simulink library "PC_Simulator_Lib"  (Simulink 8.2)
settings: Solver=ode45  StartTime=0.0  StopTime=10.0  RelTol=1e-3
values from neighbouring files (symbols this model uses):
  data = [r1 r2 r3 r4 L1 L2 L3 L4]    [strasse_Bedatung_HNI_ITI.m]
  distSameLane = 60    [InitialisationsEnv.m]
  eng_speed = [0 60 120 180 240 300 360 420 480 540 600 660 ... (101 elements, 1x101)]    [engine_table.mat]    (also in motor_parameter_calc.m = omega)
  Heading_init = 0    [Start.m]
  inertiaLateral = 25*(radiusWheel)^2    (= 4.129024)    [Start.m]
  laneWidth = 3.6    [InitialisationsEnv.m]    (also in strasse_Bedatung_HNI_ITI.m)
  omega_engine = [0.000000 150.000000 500.000000 1000.000000 1500.000000 2000.000000 2500.000000 3000.000000 3500.000000 4000.000000 4500.000000 5000.000000 5500.000000 6000.000000]    [friction_tables.m]
  omega_max = 6000    [engine_table.mat]    (also in motor_parameter_calc.m)
  omega_wheel = [0 20 40 60 80 100 122 143.7 164]    [friction_tables.m]
  para_Fellow_8_Points = ADAS.Fellow_8_Points    [ADAS_parameters.m]
  position_start_x = [x1 x2 x3 x4 x5 x6 x7]    [strasse_Bedatung_HNI_ITI.m]
  position_start_y = [y1 y2 y3 y4 y5 y6 y7]    [strasse_Bedatung_HNI_ITI.m]
  rad3rdLine = 57.2    [InitialisationsEnv.m]    (also in strasse_Bedatung_HNI_ITI.m)
  radiusWheel = 16*2.54/100    (= 0.4064)    [Start.m]
  s_values = [S1 S2 S3 S4 S5 S6 S7]    [strasse_Bedatung_HNI_ITI.m]
  segmentLimits = [segment1EndThirdLine                   segment2EndThirdLine                   segment3EndThirdLine                   segment4EndThirdLine                   segment5EndThirdLine                   segment6EndThirdLine                   segment7EndThirdLine                   segment8EndThirdLine                   ]    [InitialisationsEnv.m]    (also in strasse_Bedatung_HNI_ITI.m)
  setPosT = [-1.8 -5.4 -1.8 -5.4 -1.8 -5.4 -1.8 -5.4 -1.8 -5.4]    [InitialisationsEnv.m]
  torque = [297.089227105 300.997600937 304.800343044 308.497453426 312.088932082 315.574779014 318.95499422 322.229577701 325.398529457 328.461849487 331.419537793 334.271594373 ... (101 elements, 1x101)]    [engine_table.mat]    (also in motor_parameter_calc.m = g)
  Torque_lost = [0.000000 -8.777780 -15.000000 -26.800000 -29.600000 -32.700000 -35.900000 -39.300000 -42.800000 -46.500000 -50.300000 -54.300000 -58.500000 -62.800000 ]*0.6    [friction_tables.m]
  Torque_lost_wheel = [0.8 0.8 0.75 0.7 0.4 0.3 0.2 0.07 0.07]*0.2    [friction_tables.m]
  X_init = 0    [Start.m]
  Y_init = 1.8    [Start.m]
  Z_init = 0    [Start.m]
undefined symbols (not defined in the file or in its folder): Acc_Pedal, ADAS, Brake_Pedal, Joystick, Newton, Para, Raphson, Standard_Devices, Steering_Wheel_Angle, UDP_Protocol
libraries: simulink x43, rtwinlib x7, dspnetwork x2, simulink_extras x1, vrlib x1
(part 4 of 13)

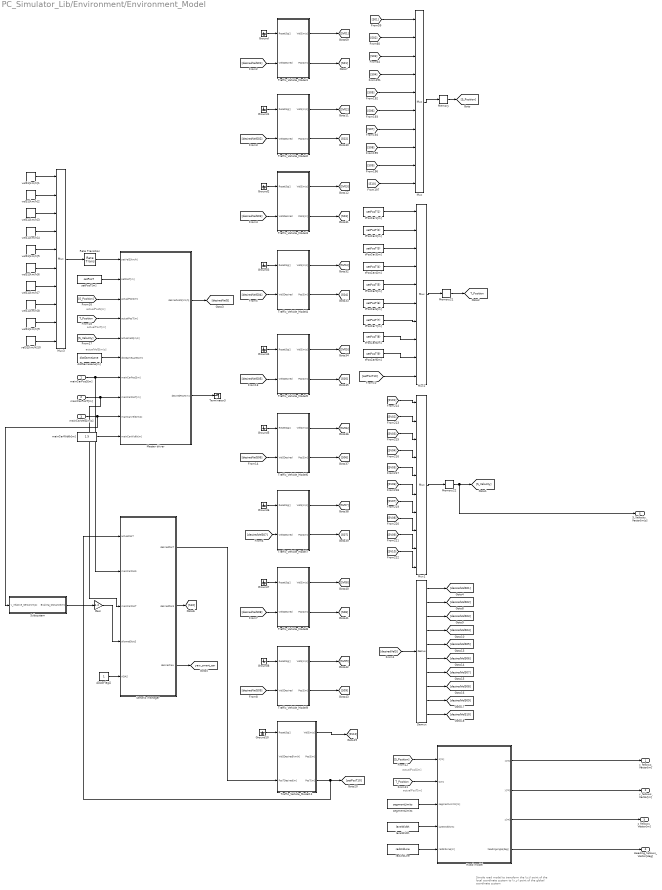
== system PC_Simulator_Lib/Environment/Environment_Model ==
  note: actualPosS[m]
  note: actualPosT[m]
  note: actualVelS[m/s]
  note: Simple road model to transform the (s,t) point of the
      | local coordinate system to (x,y) point of the global
      | coordinate system
  note: actualPosT[m]
  note: actualPosS[m]
  mainCarPosS[m] : Inport
  mainCarPosT[m] : Inport  Port=2
  mainCarVelS[m/s] : Inport  Port=3
  ADASFlag[] : Constant
  Demux : Demux  Outputs=10
  Gain : Gain  Gain=1.2
  Ground{,1..8,10} (10 alike) : Ground
  Master driver : Subsystem
  Memory : Memory
  Memory21 : Memory
  Memory22 : Memory
  Mux{,1..3} (4 alike) : Mux  Inputs=10
  Rate Transition : RateTransition
  Road model : Subsystem  Description=Simple road model to transform the (s,t) point of the local coordinate system to (x,y) point of the global coordinate system
  Senario manager : MATLAB Function  TreatAsAtomicUnit=on
  Subsystem : Subsystem
  Terminator3 : Terminator
  Traffic_Vehicle_Model1 : Subsystem
  Traffic_Vehicle_Model11 : Subsystem
  Traffic_Vehicle_Model2 : Subsystem
  Traffic_Vehicle_Model3 : Subsystem
  Traffic_Vehicle_Model4 : Subsystem
  Traffic_Vehicle_Model5 : Subsystem
  Traffic_Vehicle_Model6 : Subsystem
  Traffic_Vehicle_Model7 : Subsystem
  Traffic_Vehicle_Model8 : Subsystem
  Traffic_Vehicle_Model9 : Subsystem
  distSameLane[m] : Constant  Value=distSameLane
  laneWidth : Constant  Value=laneWidth
  mainCarWidth[m] : Constant  Value=1.5
  rad3rdLine : Constant  Value=rad3rdLine
  segmentLimits : Constant  Value=segmentLimits
  setPosT[m] : Constant  Value=setPosT
  tPosCar1[m] : Constant  Value=setPosT(1)
  tPosCar2[m] : Constant  Value=setPosT(2)
  tPosCar3[m] : Constant  Value=setPosT(3)
  tPosCar4[m] : Constant  Value=setPosT(4)
  tPosCar5[m] : Constant  Value=setPosT(5)
  tPosCar6[m] : Constant  Value=setPosT(6)
  tPosCar7[m] : Constant  Value=setPosT(7)
  tPosCar8[m] : Constant  Value=setPosT(8)
  tPosCar9[m] : Constant  Value=setPosT(9)
  velS1[km/h]1 : UniformRandomNumber  Minimum=0  Maximum=100  Seed=40  SampleTime=30
  velS1[km/h]{2..10} (9 alike) : UniformRandomNumber  Minimum=0  Maximum=100  SampleTime=30
  x_fellows_Vector[m] : Outport
  y_fellows_Vector[m] : Outport  Port=2
  z_fellows_Vector[m] : Outport  Port=3
  Heading_fellows_Vector[deg] : Outport  Port=4
  S_Velocity_Vector[m|s] : Outport  Port=5
  tag scope: T_Position=global, yaw_smart_car=global
  wires:
  [setPosT10] -> Mux2/10
  tPosCar9[m]/1 -> Mux2/9
  tPosCar8[m]/1 -> Mux2/8
  tPosCar7[m]/1 -> Mux2/7
  tPosCar3[m]/1 -> Mux2/3
  tPosCar4[m]/1 -> Mux2/4
  tPosCar1[m]/1 -> Mux2/1
  tPosCar2[m]/1 -> Mux2/2
  tPosCar6[m]/1 -> Mux2/6
  tPosCar5[m]/1 -> Mux2/5
  [S05] -> Mux/5
  [S08] -> Mux/8
  [S06] -> Mux/6
  [S07] -> Mux/7
  [S09] -> Mux/9
  [S10] -> Mux/10
  [S03] -> Mux/3
  [S04] -> Mux/4
  [S02] -> Mux/2
  [S01] -> Mux/1
  Gain/1 -> Senario manager/4(allowedDistS)
  Senario manager/1(desiredPosT) -> Traffic_Vehicle_Model11/3(PosTDesired[m])
  mainCarPosS[m]/1 -> Senario manager/2(mainCarPosS), Master driver/7(mainCarPosS[m])
  Subsystem/1(Braking_Distance[m]) -> Gain/1
  Senario manager/3(desiredYaw) -> [yaw_smart_car]
  Senario manager/2(desiredPosS) -> [S10]
  ADASFlag[]/1 -> Senario manager/5(ADAS)
  Traffic_Vehicle_Model11/3(PosT[m]) -> [setPosT10], Senario manager/1(actualPosT)
  mainCarPosT[m]/1 -> Master driver/8(mainCarPosT[m]), Senario manager/3(mainCarPosT)
  Traffic_Vehicle_Model11/1(VelS[m/s]) -> [SV10]
  Ground10/1 -> Traffic_Vehicle_Model11/1(ResetSig[])
  setPosT[m]/1 -> Master driver/2(setPosT[m])
  Master driver/2(desiredPosT[m]) -> Terminator3/1
  Mux/1 -> Memory/1
  Memory/1 -> [S_Position]
  Mux2/1 -> Memory21/1
  Memory21/1 -> [T_Position]
  Mux1/1 -> Memory22/1
  Memory22/1 -> S_Velocity_Vector[m|s]/1, [S_Velocity]
  [SV01] -> Mux1/1
  [SV02] -> Mux1/2
  [SV03] -> Mux1/3
  [SV04] -> Mux1/4
  [SV05] -> Mux1/5
  [SV06] -> Mux1/6
  [SV07] -> Mux1/7
  [SV08] -> Mux1/8
  [SV09] -> Mux1/9
  [SV10] -> Mux1/10
  [S_Position] -> Master driver/3(actualPosS[m])
  [T_Position] -> Master driver/4(actualPosT[m])
  [S_Velocity] -> Master driver/5(actualVelS[m/s])
  distSameLane[m]/1 -> Master driver/6(distSameLanes[m])
  Mux3/1 -> Rate Transition/1
  Master driver/1(desiredVelS[km/h]) -> [desiredVelS]
  [desiredVelS] -> Demux/1
  Demux/1 -> [desiredVelS01]
  Demux/2 -> [desiredVelS02]
  Demux/3 -> [desiredVelS03]
  Demux/4 -> [desiredVelS04]
  Demux/5 -> [desiredVelS05]
  Demux/6 -> [desiredVelS06]
  Demux/7 -> [desiredVelS07]
  Demux/8 -> [desiredVelS08]
  Demux/9 -> [desiredVelS09]
  Demux/10 -> [desiredVelS10]
  Ground/1 -> Traffic_Vehicle_Model1/1(ResetSig[])
  Traffic_Vehicle_Model1/2(PosS[m]) -> [S01]
  Traffic_Vehicle_Model1/1(VelS[m/s]) -> [SV01]
  [desiredVelS01] -> Traffic_Vehicle_Model1/2(VelSDesired)
  Ground1/1 -> Traffic_Vehicle_Model2/1(ResetSig[])
  Traffic_Vehicle_Model2/2(PosS[m]) -> [S02]
  Traffic_Vehicle_Model2/1(VelS[m/s]) -> [SV02]
  [desiredVelS02] -> Traffic_Vehicle_Model2/2(VelSDesired)
  Ground2/1 -> Traffic_Vehicle_Model3/1(ResetSig[])
  Traffic_Vehicle_Model3/2(PosS[m]) -> [S03]
  Traffic_Vehicle_Model3/1(VelS[m/s]) -> [SV03]
  [desiredVelS03] -> Traffic_Vehicle_Model3/2(VelSDesired)
  Ground3/1 -> Traffic_Vehicle_Model4/1(ResetSig[])
  Traffic_Vehicle_Model4/2(PosS[m]) -> [S04]
  Traffic_Vehicle_Model4/1(VelS[m/s]) -> [SV04]
  [desiredVelS04] -> Traffic_Vehicle_Model4/2(VelSDesired)
  Ground4/1 -> Traffic_Vehicle_Model5/1(ResetSig[])
  Traffic_Vehicle_Model5/2(PosS[m]) -> [S05]
  Traffic_Vehicle_Model5/1(VelS[m/s]) -> [SV05]
  [desiredVelS05] -> Traffic_Vehicle_Model5/2(VelSDesired)
  Ground5/1 -> Traffic_Vehicle_Model6/1(ResetSig[])
  Traffic_Vehicle_Model6/2(PosS[m]) -> [S06]
  Traffic_Vehicle_Model6/1(VelS[m/s]) -> [SV06]
  [desiredVelS06] -> Traffic_Vehicle_Model6/2(VelSDesired)
  Ground6/1 -> Traffic_Vehicle_Model7/1(ResetSig[])
  Traffic_Vehicle_Model7/2(PosS[m]) -> [S07]
  Traffic_Vehicle_Model7/1(VelS[m/s]) -> [SV07]
  [desiredVelS07] -> Traffic_Vehicle_Model7/2(VelSDesired)
  Ground7/1 -> Traffic_Vehicle_Model8/1(ResetSig[])
  Traffic_Vehicle_Model8/2(PosS[m]) -> [S08]
  Traffic_Vehicle_Model8/1(VelS[m/s]) -> [SV08]
  [desiredVelS08] -> Traffic_Vehicle_Model8/2(VelSDesired)
  Ground8/1 -> Traffic_Vehicle_Model9/1(ResetSig[])
  Traffic_Vehicle_Model9/2(PosS[m]) -> [S09]
  Traffic_Vehicle_Model9/1(VelS[m/s]) -> [SV09]
  [desiredVelS09] -> Traffic_Vehicle_Model9/2(VelSDesired)
  Road model/4(headingAngle[deg]) -> Heading_fellows_Vector[deg]/1
  Road model/2(y[m]) -> y_fellows_Vector[m]/1
  Road model/1(x[m]) -> x_fellows_Vector[m]/1
  Road model/3(z[m]) -> z_fellows_Vector[m]/1
  velS1[km/h]2/1 -> Mux3/2
  velS1[km/h]4/1 -> Mux3/4
  [S_Position] -> Road model/1(s[m])
  [T_Position] -> Road model/2(t[m])
  velS1[km/h]1/1 -> Mux3/1
  rad3rdLine/1 -> Road model/5(rad3rdLine[m])
  laneWidth/1 -> Road model/4(laneWidth[m])
  mainCarWidth[m]/1 -> Master driver/10(mainCarWidth[m])
  segmentLimits/1 -> Road model/3(segmentLimits[m])
  velS1[km/h]9/1 -> Mux3/9
  velS1[km/h]8/1 -> Mux3/8
  velS1[km/h]3/1 -> Mux3/3
  velS1[km/h]7/1 -> Mux3/7
  velS1[km/h]6/1 -> Mux3/6
  Rate Transition/1 -> Master driver/1(setVelS[km/h])
  velS1[km/h]5/1 -> Mux3/5
  velS1[km/h]10/1 -> Mux3/10
  mainCarVelS[m/s]/1 -> Master driver/9(mainCarVelS[m/s]), Subsystem/1(v_relative_Sensor[m|s])

== system PC_Simulator_Lib/Environment/Maping_Input  ==
  Feedback : Inport
  Bus Selector10 : BusSelector  OutputSignals=Vehicle_Dynamics.position_CoG.x_CoG[m],Vehicle_Dynamics.position_CoG.y_CoG[m],Vehicle_Dynamics.Vx_COG[m|s]
  Gain : Gain  Gain=180/pi
  Strasse_xy : Subsystem
  mainCarPosS[m] : Outport
  mainCarPosT[m] : Outport  Port=2
  mainCarVelS[m/s] : Outport  Port=3
  Heating_Angle_Road_under_VUT[deg] : Outport  Port=4
  wires:
  Bus Selector10/1 -> Strasse_xy/1(x[m])  "<x_CoG[m]>"
  Bus Selector10/2 -> Strasse_xy/2(y[m])  "<y_CoG[m]>"
  Strasse_xy/2(t[m]) -> mainCarPosT[m]/1  "t_VUT[m]"
  Strasse_xy/1(s[m]) -> mainCarPosS[m]/1  "s_VUT[m]"
  Feedback/1 -> Bus Selector10/1
  Bus Selector10/3 -> mainCarVelS[m/s]/1  "<Vx_COG[m|s]>"
  Strasse_xy/3(Heading_angle[rad]) -> Gain/1
  Gain/1 -> Heating_Angle_Road_under_VUT[deg]/1

== system PC_Simulator_Lib/Environment/Maping_Output  ==
  x_fellows_Vector[m] : Inport
  y_fellows_Vector[m] : Inport  Port=2
  z_fellows_Vector[m] : Inport  Port=3
  Heading_fellows_Vector[deg] : Inport  Port=4
  S_Velocity_Vector[m|s] : Inport  Port=5
  T_VUT[m] : Inport  Port=6
  Heating_Angle_Road_under_VUT[deg] : Inport  Port=7
  Bus Creator : BusCreator  Inputs=11
  Bus Creator{1,3..11} (10 alike) : BusCreator  Inputs=5
  Bus Creator2 : BusCreator  Inputs=2
  Bus Selector : BusSelector  OutputSignals=x_fellows_vector.x_fellow1[m],y_fellows_vector.y_fellow1[m],z_fellows_vector.z_fellow1[m],Heading_fellows_vector.Heading_fellow1[deg],velocity_fellows_vector[m|s].velocity_fellow1[m|s]
  Bus Selector1 : BusSelector  OutputSignals=x_fellows_vector.x_fellow2[m],y_fellows_vector.y_fellow2[m],z_fellows_vector.z_fellow2[m],Heading_fellows_vector.Heading_fellow2[deg],velocity_fellows_vector[m|s].velocity_fellow2[m|s]
  Bus Selector2 : BusSelector  OutputSignals=x_fellows_vector.x_fellow3[m],y_fellows_vector.y_fellow3[m],z_fellows_vector.z_fellow3[m],Heading_fellows_vector.Heading_fellow3[deg],velocity_fellows_vector[m|s].velocity_fellow3[m|s]
  Bus Selector3 : BusSelector  OutputSignals=x_fellows_vector.x_fellow4[m],y_fellows_vector.y_fellow4[m],z_fellows_vector.z_fellow4[m],Heading_fellows_vector.Heading_fellow4[deg],velocity_fellows_vector[m|s].velocity_fellow4[m|s]
  Bus Selector4 : BusSelector  OutputSignals=x_fellows_vector.x_fellow5[m],y_fellows_vector.y_fellow5[m],z_fellows_vector.z_fellow5[m],Heading_fellows_vector.Heading_fellow5[deg],velocity_fellows_vector[m|s].velocity_fellow5[m|s]
  Bus Selector5 : BusSelector  OutputSignals=x_fellows_vector.x_fellow6[m],y_fellows_vector.y_fellow6[m],z_fellows_vector.z_fellow6[m],Heading_fellows_vector.Heading_fellow6[deg],velocity_fellows_vector[m|s].velocity_fellow6[m|s]
  Bus Selector6 : BusSelector  OutputSignals=x_fellows_vector.x_fellow7[m],y_fellows_vector.y_fellow7[m],z_fellows_vector.z_fellow7[m],Heading_fellows_vector.Heading_fellow7[deg],velocity_fellows_vector[m|s].velocity_fellow7[m|s]
  Bus Selector7 : BusSelector  OutputSignals=x_fellows_vector.x_fellow8[m],y_fellows_vector.y_fellow8[m],z_fellows_vector.z_fellow8[m],Heading_fellows_vector.Heading_fellow8[deg],velocity_fellows_vector[m|s].velocity_fellow8[m|s]
  Bus Selector8 : BusSelector  OutputSignals=x_fellows_vector.x_fellow9[m],y_fellows_vector.y_fellow9[m],z_fellows_vector.z_fellow9[m],Heading_fellows_vector.Heading_fellow9[deg],velocity_fellows_vector[m|s].velocity_fellow9[m|s]
  Bus Selector9 : BusSelector  OutputSignals=x_fellows_vector.x_fellow10[m],y_fellows_vector.y_fellow10[m],z_fellows_vector.z_fellow10[m],Heading_fellows_vector.Heading_fellow10[deg],velocity_fellows_vector[m|s].velocity_fellow10[m|s]
  Subsystem : Subsystem
  Out1 : Outport
  wires:
  Bus Creator/1 -> Out1/1  "Environment"
  Bus Selector/2 -> Bus Creator1/2  "<y_fellow1[m]>"
  Bus Selector/1 -> Bus Creator1/1  "<x_fellow1[m]>"
  Bus Selector/4 -> Bus Creator1/4  "<Heading_fellow1[deg]>"
  Bus Creator1/1 -> Bus Creator/2  "fellow_car_1"
  Bus Creator2/1 -> Bus Creator/1  "Main_Vehicle"
  Bus Selector/3 -> Bus Creator1/3  "<z_fellow1[m]>"
  x_fellows_Vector[m]/1 -> Subsystem/1(x_fellows_Vector[m])
  y_fellows_Vector[m]/1 -> Subsystem/2(y_fellows_Vector[m])
  z_fellows_Vector[m]/1 -> Subsystem/3(z_fellows_Vector[m])
  Heading_fellows_Vector[deg]/1 -> Subsystem/4(Heading_fellows_Vector[deg])
  Subsystem/1(Fellows_Pos_Oriantation_Bus) -> Bus Selector9/1, Bus Selector8/1, Bus Selector7/1, Bus Selector6/1, Bus Selector5/1, Bus Selector4/1, Bus Selector3/1, Bus Selector2/1, Bus Selector1/1, Bus Selector/1
  Bus Selector1/2 -> Bus Creator3/2  "<y_fellow2[m]>"
  Bus Selector1/1 -> Bus Creator3/1  "<x_fellow2[m]>"
  Bus Selector1/4 -> Bus Creator3/4  "<Heading_fellow2[deg]>"
  Bus Creator3/1 -> Bus Creator/3  "fellow_car_2"
  Bus Selector1/3 -> Bus Creator3/3  "<z_fellow2[m]>"
  Bus Selector2/2 -> Bus Creator4/2  "<y_fellow3[m]>"
  Bus Selector2/1 -> Bus Creator4/1  "<x_fellow3[m]>"
  Bus Selector2/4 -> Bus Creator4/4  "<Heading_fellow3[deg]>"
  Bus Creator4/1 -> Bus Creator/4  "fellow_car_3"
  Bus Selector2/3 -> Bus Creator4/3  "<z_fellow3[m]>"
  Bus Selector3/2 -> Bus Creator5/2  "<y_fellow4[m]>"
  Bus Selector3/1 -> Bus Creator5/1  "<x_fellow4[m]>"
  Bus Selector3/4 -> Bus Creator5/4  "<Heading_fellow4[deg]>"
  Bus Creator5/1 -> Bus Creator/5  "fellow_car_4"
  Bus Selector3/3 -> Bus Creator5/3  "<z_fellow4[m]>"
  Bus Selector4/2 -> Bus Creator6/2  "<y_fellow5[m]>"
  Bus Selector4/1 -> Bus Creator6/1  "<x_fellow5[m]>"
  Bus Selector4/4 -> Bus Creator6/4  "<Heading_fellow5[deg]>"
  Bus Creator6/1 -> Bus Creator/6  "fellow_car_5"
  Bus Selector4/3 -> Bus Creator6/3  "<z_fellow5[m]>"
  Bus Creator7/1 -> Bus Creator/7  "fellow_car_6"
  Bus Creator8/1 -> Bus Creator/8  "fellow_car_7"
  Bus Creator9/1 -> Bus Creator/9  "fellow_car_8"
  Bus Creator10/1 -> Bus Creator/10  "fellow_car_9"
  Bus Creator11/1 -> Bus Creator/11  "fellow_car_10"
  Bus Selector5/3 -> Bus Creator7/3  "<z_fellow6[m]>"
  Bus Selector5/4 -> Bus Creator7/4  "<Heading_fellow6[deg]>"
  Bus Selector5/2 -> Bus Creator7/2  "<y_fellow6[m]>"
  Bus Selector5/1 -> Bus Creator7/1  "<x_fellow6[m]>"
  Bus Selector6/2 -> Bus Creator8/2  "<y_fellow7[m]>"
  Bus Selector6/4 -> Bus Creator8/4  "<Heading_fellow7[deg]>"
  Bus Selector6/1 -> Bus Creator8/1  "<x_fellow7[m]>"
  Bus Selector6/3 -> Bus Creator8/3  "<z_fellow7[m]>"
  Bus Selector7/2 -> Bus Creator9/2  "<y_fellow8[m]>"
  Bus Selector7/1 -> Bus Creator9/1  "<x_fellow8[m]>"
  Bus Selector7/3 -> Bus Creator9/3  "<z_fellow8[m]>"
  Bus Selector7/4 -> Bus Creator9/4  "<Heading_fellow8[deg]>"
  Bus Selector8/2 -> Bus Creator10/2  "<y_fellow9[m]>"
  Bus Selector8/1 -> Bus Creator10/1  "<x_fellow9[m]>"
  Bus Selector8/4 -> Bus Creator10/4  "<Heading_fellow9[deg]>"
  Bus Selector8/3 -> Bus Creator10/3  "<z_fellow9[m]>"
  Bus Selector9/4 -> Bus Creator11/4  "<Heading_fellow10[deg]>"
  Bus Selector9/3 -> Bus Creator11/3  "<z_fellow10[m]>"
  Bus Selector9/1 -> Bus Creator11/1  "<x_fellow10[m]>"
  Bus Selector9/2 -> Bus Creator11/2  "<y_fellow10[m]>"
  T_VUT[m]/1 -> Bus Creator2/1
  S_Velocity_Vector[m|s]/1 -> Subsystem/5(S_Velocity_Vector[m|s])
  Bus Selector/5 -> Bus Creator1/5  "<velocity_fellow1[m|s]>"
  Bus Selector1/5 -> Bus Creator3/5  "<velocity_fellow2[m|s]>"
  Bus Selector2/5 -> Bus Creator4/5  "<velocity_fellow3[m|s]>"
  Bus Selector3/5 -> Bus Creator5/5  "<velocity_fellow4[m|s]>"
  Bus Selector4/5 -> Bus Creator6/5  "<velocity_fellow5[m|s]>"
  Bus Selector5/5 -> Bus Creator7/5  "<velocity_fellow6[m|s]>"
  Bus Selector6/5 -> Bus Creator8/5  "<velocity_fellow7[m|s]>"
  Bus Selector7/5 -> Bus Creator9/5  "<velocity_fellow8[m|s]>"
  Bus Selector8/5 -> Bus Creator10/5  "<velocity_fellow9[m|s]>"
  Bus Selector9/5 -> Bus Creator11/5  "<velocity_fellow10[m|s]>"
  Heating_Angle_Road_under_VUT[deg]/1 -> Bus Creator2/2  "Heating_Angle_Road_under_VUT[deg]"

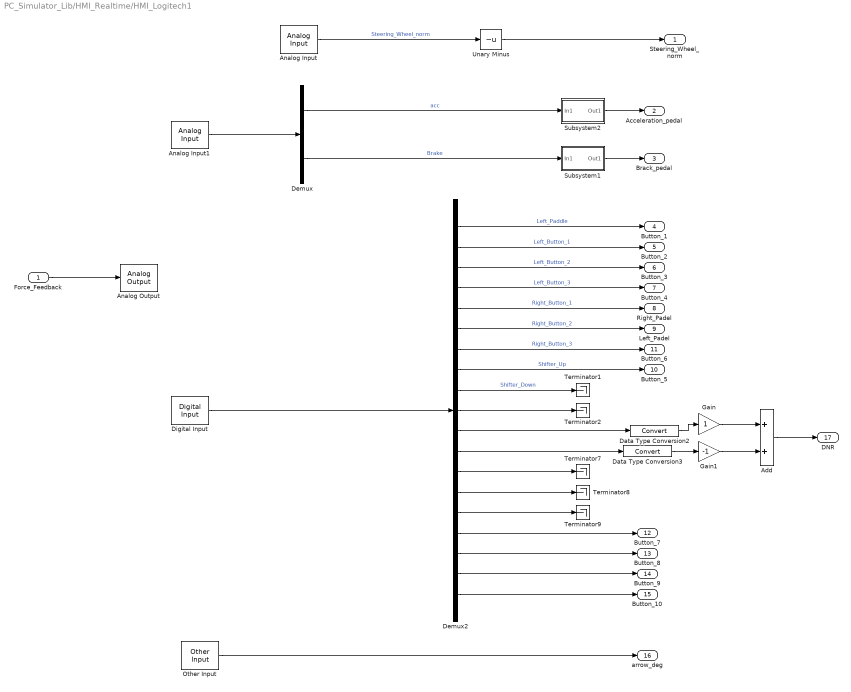
== system PC_Simulator_Lib/HMI_Realtime/HMI_Logitech1 ==
  Force_Feedback : Inport
  Add : Sum
  Analog Input : rtwinlib/Analog Input  SampleTime=-1  MaxMissedTicks=[]  ShowMissedTicks=off  YieldWhenWaiting=off  DrvName=Standard_Devices/Joystick  DrvAddress=1  DrvOptions=zeros(1,0)  Channels=1  RangeMode=2  VoltRange=1  DataType=1
      settings: AttributesFormatString=Standard Devices\nJoystick [1h]
  Analog Input1 : rtwinlib/Analog Input  SampleTime=-1  MaxMissedTicks=[]  ShowMissedTicks=off  YieldWhenWaiting=off  DrvName=Standard_Devices/Joystick  DrvAddress=1  DrvOptions=zeros(1,0)  Channels=2:3  RangeMode=3  VoltRange=1  DataType=1
      settings: AttributesFormatString=Standard Devices\nJoystick [1h]
  Analog Output : rtwinlib/Analog Output  SampleTime=0.001  MaxMissedTicks=[]  ShowMissedTicks=off  YieldWhenWaiting=off  DrvName=Standard_Devices/Joystick  DrvAddress=1  DrvOptions=zeros(1,0)  Channels=1  RangeMode=1  VoltRange=1  InitialValue=[]  FinalValue=[]
      settings: AttributesFormatString=Standard Devices\nJoystick [1h]
  Data Type Conversion2 : DataTypeConversion
  Data Type Conversion3 : DataTypeConversion
  Demux : Demux  Outputs=2
  Demux2 : Demux  Outputs=19
  Digital Input : rtwinlib/Digital Input  SampleTime=-1  MaxMissedTicks=[]  ShowMissedTicks=off  YieldWhenWaiting=off  DrvName=Standard_Devices/Joystick  DrvAddress=1  DrvOptions=zeros(1,0)  Channels=1:19  BitMode=1  DataType=1
      settings: AttributesFormatString=Standard Devices\nJoystick [1h]
  Gain : Gain
  Gain1 : Gain  Gain=-1
  Other Input : rtwinlib/Other Input  SampleTime=-1  MaxMissedTicks=[]  ShowMissedTicks=off  YieldWhenWaiting=off  DrvName=Standard_Devices/Joystick  DrvAddress=1  DrvOptions=zeros(1,0)  Channels=1  OptParam=0  DataType=1
      settings: AttributesFormatString=Standard Devices\nJoystick [1h]
  Subsystem1 : Subsystem
  Subsystem2 : Subsystem
  Terminator{1..2,7..9} (5 alike) : Terminator
  Unary Minus : UnaryMinus
  Steering_Wheel_norm : Outport
  Acceleration_pedal : Outport  Port=2
  Brack_pedal : Outport  Port=3
  Button_1 : Outport  Port=4
  Button_2 : Outport  Port=5
  Button_3 : Outport  Port=6
  Button_4 : Outport  Port=7
  Right_Padel : Outport  Port=8
  Left_Padel : Outport  Port=9
  Button_5 : Outport  Port=10
  Button_6 : Outport  Port=11
  Button_7 : Outport  Port=12
  Button_8 : Outport  Port=13
  Button_9 : Outport  Port=14
  Button_10 : Outport  Port=15
  arrow_deg : Outport  Port=16
  DNR : Outport  Port=17
  wires:
  Demux2/12 -> Data Type Conversion3/1
  Demux2/11 -> Data Type Conversion2/1
  Demux2/10 -> Terminator2/1
  Demux2/9 -> Terminator1/1  "Shifter_Down"
  Digital Input/1 -> Demux2/1
  Demux/1 -> Subsystem2/1(In1)  "acc"
  Demux/2 -> Subsystem1/1(In1)  "Brake"
  Analog Input/1 -> Unary Minus/1  "Steering_Wheel_norm"
  Subsystem2/1(Out1) -> Acceleration_pedal/1
  Subsystem1/1(Out1) -> Brack_pedal/1
  Demux2/1 -> Button_1/1  "Left_Paddle"
  Demux2/2 -> Button_2/1  "Left_Button_1"
  Demux2/3 -> Button_3/1  "Left_Button_2"
  Demux2/4 -> Button_4/1  "Left_Button_3"
  Demux2/5 -> Right_Padel/1  "Right_Button_1"
  Demux2/6 -> Left_Padel/1  "Right_Button_2"
  Demux2/7 -> Button_6/1  "Right_Button_3"
  Demux2/8 -> Button_5/1  "Shifter_Up"
  Demux2/16 -> Button_7/1
  Demux2/17 -> Button_8/1
  Demux2/18 -> Button_9/1
  Demux2/19 -> Button_10/1
  Other Input/1 -> arrow_deg/1
  Unary Minus/1 -> Steering_Wheel_norm/1
  Gain/1 -> Add/1
  Gain1/1 -> Add/2
  Add/1 -> DNR/1
  Data Type Conversion2/1 -> Gain/1
  Data Type Conversion3/1 -> Gain1/1
  Demux2/13 -> Terminator7/1
  Demux2/14 -> Terminator8/1
  Demux2/15 -> Terminator9/1
  Analog Input1/1 -> Demux/1
  Force_Feedback/1 -> Analog Output/1

== system PC_Simulator_Lib/HMI_Realtime/Maping_Output ==
  Steering_wheel_norm : Inport
  Acc_Pedal_norm : Inport  Port=2
  Brake_Pedal_norm : Inport  Port=3
  ACC_Plus : Inport  Port=4
  ACC_Minus : Inport  Port=5
  ACC_Stop : Inport  Port=6
  ACC_Resume : Inport  Port=7
  Emergency_Brake_Button : Inport  Port=8
  Pilot_Button : Inport  Port=9
  Time_Gap_Mode_Switching : Inport  Port=10
  Emergency_Steering_Button : Inport  Port=11
  DNR : Inport  Port=12
  Bus Creator : BusCreator  Inputs=12
  Data Type Conversion{,1..7} (8 alike) : DataTypeConversion
  Gain{,1..11} (12 alike) : Gain
  Out1 : Outport
  wires:
  Bus Creator/1 -> Out1/1  "Driver_Interface"
  DNR/1 -> Gain3/1
  Acc_Pedal_norm/1 -> Gain1/1
  Brake_Pedal_norm/1 -> Gain2/1
  Steering_wheel_norm/1 -> Gain/1
  ACC_Plus/1 -> Data Type Conversion/1
  ACC_Minus/1 -> Data Type Conversion1/1
  ACC_Resume/1 -> Data Type Conversion3/1
  ACC_Stop/1 -> Data Type Conversion2/1
  Gain/1 -> Bus Creator/1  "Steering_wheel_norm"
  Gain1/1 -> Bus Creator/2  "Acc_Pedal_norm"
  Gain2/1 -> Bus Creator/3  "Brake_Pedal_norm"
  Gain3/1 -> Bus Creator/4  "DNR"
  Gain4/1 -> Bus Creator/5  "ACC_Plus_Button"
  Gain5/1 -> Bus Creator/6  "ACC_Minus_Button"
  Gain6/1 -> Bus Creator/7  "ACC_Stop_Button"
  Gain7/1 -> Bus Creator/8  "ACC_Resume_Button"
  Data Type Conversion/1 -> Gain4/1
  Data Type Conversion1/1 -> Gain5/1
  Data Type Conversion2/1 -> Gain6/1
  Data Type Conversion3/1 -> Gain7/1
  Data Type Conversion4/1 -> Gain8/1
  Gain8/1 -> Bus Creator/9  "Time_Gap_Mode_Switching_Button"
  Time_Gap_Mode_Switching/1 -> Data Type Conversion4/1
  Data Type Conversion5/1 -> Gain9/1
  Gain9/1 -> Bus Creator/10  "Pilot_Button"
  Pilot_Button/1 -> Data Type Conversion5/1
  Data Type Conversion6/1 -> Gain10/1
  Emergency_Brake_Button/1 -> Data Type Conversion6/1
  Gain10/1 -> Bus Creator/11  "Emergency_Brake_Button"
  Data Type Conversion7/1 -> Gain11/1
  Gain11/1 -> Bus Creator/12  "Emergency_Steering_Button"
  Emergency_Steering_Button/1 -> Data Type Conversion7/1

== system PC_Simulator_Lib/HMI_Realtime/steering wheel controller ==
  wheel_angle_actual_deg[-450 450] : Inport
  wheel_angle_desired_deg[-450 450] : Inport  Port=2
  controller_mod : Inport  Port=3
  1-D Lookup Table : Lookup_n-D  NumberOfTableDimensions=1  BreakpointsForDimension1=[0 5 10 15 20 30 40 50 60 70 90 120 180 300 400 450]  Table="[0 0  0.2 0.25 0.3 0.35 0.4 0.45 0.5 0.6 0.7 0.75 0.8 0.9 1 1]"  InternalRulePriority=Speed  RndMeth=Simplest  InputSameDT=on
  Abs : Abs
  Compare To Constant3 : simulink/Logic and Bit Operations/Compare To Constant  relop===  const=1  OutDataTypeStr=boolean
  Constant2 : Constant  Value=0
  Gain2 : Gain  Gain=-1
  Product : Product
  Saturation2 : Saturate  UpperLimit=450  LowerLimit=-450
  Saturation3 : Saturate  UpperLimit=450  LowerLimit=-450
  Sign : Signum
  Subtract1 : Sum  Inputs=+-
  Switch2 : Switch  Criteria=u2 > Threshold
  Out1 : Outport
  wires:
  Product/1 -> Out1/1
  Saturation3/1 -> Subtract1/1
  Compare To Constant3/1 -> Switch2/2
  controller_mod/1 -> Compare To Constant3/1
  Constant2/1 -> Switch2/3
  Switch2/1 -> Saturation3/1
  wheel_angle_desired_deg[-450 450]/1 -> Switch2/1
  Abs/1 -> 1-D Lookup Table/1
  Gain2/1 -> Product/2
  Sign/1 -> Gain2/1
  1-D Lookup Table/1 -> Product/1
  Subtract1/1 -> Sign/1, Abs/1
  wheel_angle_actual_deg[-450 450]/1 -> Saturation2/1
  Saturation2/1 -> Subtract1/2

== system PC_Simulator_Lib/HMI_Realtime_normal_mode/HMI_Logitech ==
  Add : Sum
  Data Type Conversion2 : DataTypeConversion
  Data Type Conversion3 : DataTypeConversion
  Demux : Demux  Outputs=5
  Demux2 : Demux  Outputs=19
  Gain : Gain
  Gain1 : Gain  Gain=-1
  Joystick Input : vrlib/Joystick Input  joyid=1  adjustports=on  forcefeed=off
  Subsystem2 : Subsystem
  Subsystem3 : Subsystem
  Terminator{1..2,5..9} (7 alike) : Terminator
  Unary Minus : UnaryMinus
  Steering_Wheel_norm : Outport
  Acceleration_pedal : Outport  Port=2
  Brack_pedal : Outport  Port=3
  Button_1 : Outport  Port=4
  Button_2 : Outport  Port=5
  Button_3 : Outport  Port=6
  Button_4 : Outport  Port=7
  Right_Padel : Outport  Port=8
  Left_Padel : Outport  Port=9
  Button_5 : Outport  Port=10
  Button_6 : Outport  Port=11
  Button_7 : Outport  Port=12
  Button_8 : Outport  Port=13
  Button_9 : Outport  Port=14
  Button_10 : Outport  Port=15
  arrow_deg : Outport  Port=16
  DNR : Outport  Port=17
  wires:
  Joystick Input/2 -> Demux2/1
  Joystick Input/1 -> Demux/1
  Demux/2 -> Subsystem2/1(In1)  "acc"
  Demux/3 -> Subsystem3/1(In1)  "Brake"
  Demux/1 -> Unary Minus/1  "Steering_Wheel_norm"
  Subsystem2/1(Out1) -> Acceleration_pedal/1
  Subsystem3/1(Out1) -> Brack_pedal/1
  Demux/4 -> Terminator1/1
  Demux/5 -> Terminator2/1
  Demux2/1 -> Button_1/1  "Left_Paddle"
  Demux2/2 -> Button_2/1  "Left_Button_1"
  Demux2/3 -> Button_3/1  "Left_Button_2"
  Demux2/4 -> Button_4/1  "Left_Button_3"
  Demux2/5 -> Right_Padel/1  "Right_Button_1"
  Demux2/6 -> Left_Padel/1  "Right_Button_2"
  Demux2/7 -> Button_6/1  "Right_Button_3"
  Demux2/8 -> Button_5/1  "Shifter_Up"
  Demux2/16 -> Button_7/1
  Demux2/17 -> Button_8/1
  Demux2/18 -> Button_9/1
  Demux2/19 -> Button_10/1
  Joystick Input/3 -> arrow_deg/1
  Gain/1 -> Add/1
  Data Type Conversion2/1 -> Gain/1
  Data Type Conversion3/1 -> Gain1/1
  Demux2/13 -> Terminator7/1
  Demux2/14 -> Terminator8/1
  Demux2/15 -> Terminator9/1
  Add/1 -> DNR/1
  Gain1/1 -> Add/2
  Demux2/12 -> Data Type Conversion3/1
  Demux2/11 -> Data Type Conversion2/1
  Demux2/10 -> Terminator6/1
  Demux2/9 -> Terminator5/1  "Shifter_Down"
  Unary Minus/1 -> Steering_Wheel_norm/1

== system PC_Simulator_Lib/HMI_Realtime_normal_mode/Maping_Output ==
  Steering_wheel_norm : Inport
  Acc_Pedal_norm : Inport  Port=2
  Brake_Pedal_norm : Inport  Port=3
  ACC_Plus : Inport  Port=4
  ACC_Minus : Inport  Port=5
  ACC_Stop : Inport  Port=6
  ACC_Resume : Inport  Port=7
  Emergency_Brake_Button : Inport  Port=8
  Pilot_Button : Inport  Port=9
  Time_Gap_Mode_Switching : Inport  Port=10
  Emergency_Steering_Button : Inport  Port=11
  DNR : Inport  Port=12
  Bus Creator : BusCreator  Inputs=12
  Data Type Conversion{,1..7} (8 alike) : DataTypeConversion
  Gain{,1..11} (12 alike) : Gain
  Out1 : Outport
  wires:
  Bus Creator/1 -> Out1/1  "Driver_Interface"
  DNR/1 -> Gain3/1
  Acc_Pedal_norm/1 -> Gain1/1
  Brake_Pedal_norm/1 -> Gain2/1
  Steering_wheel_norm/1 -> Gain/1
  ACC_Plus/1 -> Data Type Conversion/1
  ACC_Minus/1 -> Data Type Conversion1/1
  ACC_Resume/1 -> Data Type Conversion3/1
  ACC_Stop/1 -> Data Type Conversion2/1
  Gain/1 -> Bus Creator/1  "Steering_wheel_norm"
  Gain1/1 -> Bus Creator/2  "Acc_Pedal_norm"
  Gain2/1 -> Bus Creator/3  "Brake_Pedal_norm"
  Gain3/1 -> Bus Creator/4  "DNR"
  Gain4/1 -> Bus Creator/5  "ACC_Plus_Button"
  Gain5/1 -> Bus Creator/6  "ACC_Minus_Button"
  Gain6/1 -> Bus Creator/7  "ACC_Stop_Button"
  Gain7/1 -> Bus Creator/8  "ACC_Resume_Button"
  Data Type Conversion/1 -> Gain4/1
  Data Type Conversion1/1 -> Gain5/1
  Data Type Conversion2/1 -> Gain6/1
  Data Type Conversion3/1 -> Gain7/1
  Data Type Conversion4/1 -> Gain8/1
  Gain8/1 -> Bus Creator/9  "Time_Gap_Mode_Switching_Button"
  Time_Gap_Mode_Switching/1 -> Data Type Conversion4/1
  Data Type Conversion5/1 -> Gain9/1
  Gain9/1 -> Bus Creator/10  "Pilot_Button"
  Pilot_Button/1 -> Data Type Conversion5/1
  Data Type Conversion6/1 -> Gain10/1
  Emergency_Brake_Button/1 -> Data Type Conversion6/1
  Gain10/1 -> Bus Creator/11  "Emergency_Brake_Button"
  Data Type Conversion7/1 -> Gain11/1
  Gain11/1 -> Bus Creator/12  "Emergency_Steering_Button"
  Emergency_Steering_Button/1 -> Data Type Conversion7/1

== system PC_Simulator_Lib/Vehicle dynamics/Forces_transformation ==
  note: this block is to produce the whole
      | forces and moments that is applied
      | on the car transformed to the vehicle
      | center of gravity CG
  velocity_of_car_absolute : Inport
  Slip_angle_of_velocity : Inport  Port=2
  Forces_on_x_from_wheel_mux(4) : Inport  Port=3
  Forces_on_y_from_wheel_mux(4) : Inport  Port=4
  Forces_on_z_from_wheel_mux(4) : Inport  Port=5
  Length_suspention(4) : Inport  Port=6
  Z0_mux(4) : Inport  Port=7
  Demux : Demux
  Force_of_Aerodynamics : Subsystem
  Moment _about _Z_axis_calculation : Subsystem
  Moment _about _x_axis_calculation : Subsystem
  Moment _about _y_axis_calculation : Subsystem
  Z1-->angles : Subsystem
  force acting in X direction : Subsystem
  force acting in Y direction : Subsystem
  force acting in Z direction : Subsystem
  inclination_effect_on_mass : Subsystem
  Force_acting_on_CG_in_x : Outport
  Force_acting_on_CG_in_Y : Outport  Port=2
  Moment _about _Z_axis : Outport  Port=3
  Force_acting_on_CG_in_z : Outport  Port=4
  Moment _about _X_axis : Outport  Port=5
  Moment _about _Y_axis : Outport  Port=6
  Mass*gravity_in_Z : Outport  Port=7
  wires:
  force acting in X direction/1(Force_acting_on_CG_in_x) -> Force_acting_on_CG_in_x/1
  force acting in Y direction/1(Force_acting_on_CG_in_Y) -> Force_acting_on_CG_in_Y/1
  Moment _about _Z_axis_calculation/1(Moment _about _Z_axis) -> Moment _about _Z_axis/1
  velocity_of_car_absolute/1 -> Force_of_Aerodynamics/1(velocity_of_car_absolut)
  Slip_angle_of_velocity/1 -> Force_of_Aerodynamics/2(Slip_angle_of_velocity)
  Forces_on_x_from_wheel_mux(4)/1 -> force acting in X direction/1(Forces_Acting_In_X_Wheel), Moment _about _Z_axis_calculation/1(Forces_Acting_in_X_Wheels), Moment _about _y_axis_calculation/2(Forces_X_Wheels)
  Forces_on_y_from_wheel_mux(4)/1 -> Moment _about _x_axis_calculation/2(Forces_Y_Wheels), Moment _about _Z_axis_calculation/2(Forces_Acting_in_Y_Wheels), force acting in Y direction/1(Forces_Acting_In_Y_Wheels)
  Forces_on_z_from_wheel_mux(4)/1 -> force acting in Z direction/1(Forces_Z_Wheel), Moment _about _x_axis_calculation/1(Forces_Z_Wheels), Moment _about _y_axis_calculation/1(Forces_Z_Wheels)
  force acting in Z direction/1(Force_acting_on_CG_in_z) -> Force_acting_on_CG_in_z/1
  Moment _about _x_axis_calculation/1(Moment _about _X_axis1) -> Moment _about _X_axis/1
  inclination_effect_on_mass/1(FZ_due_to_mass) -> force acting in Z direction/2(Force_Mass_Z), Mass*gravity_in_Z/1
  Moment _about _y_axis_calculation/1(Moment _about _Y_axis2) -> Moment _about _Y_axis/1
  Demux/1 -> Moment _about _x_axis_calculation/3(Hight_Front_Left), Moment _about _y_axis_calculation/3(Hight_Front_Left)
  Demux/2 -> Moment _about _x_axis_calculation/4(Hight_Front_Right), Moment _about _y_axis_calculation/4(Hight_Front_Right)
  Demux/3 -> Moment _about _x_axis_calculation/5(Hight_Rear_Left), Moment _about _y_axis_calculation/5(Hight_Rear_Left)
  Demux/4 -> Moment _about _x_axis_calculation/6(Hight_Rear_Right), Moment _about _y_axis_calculation/6(Hight_Rear_Right)
  Force_of_Aerodynamics/1(Force_of_aerodynamics_in_X) -> force acting in X direction/3(Force_in_x_air)
  Length_suspention(4)/1 -> Demux/1
  Z1-->angles/2(Pitch_angel(z1)) -> inclination_effect_on_mass/2(Pitch_angel(z1))
  Z1-->angles/1(Roll_angel(z1)1) -> inclination_effect_on_mass/1(Roll_angle(z1))
  inclination_effect_on_mass/2(Fx_due_to_mass) -> force acting in X direction/2(Force_acting_in_x_from_mass)
  inclination_effect_on_mass/3(Fy_due_to_mass) -> force acting in Y direction/2(Force_From_Mass_Y)
  Z0_mux(4)/1 -> Z1-->angles/1(Z1(4))

== system PC_Simulator_Lib/Vehicle dynamics/Horizontal_Dyn ==
  note: through this block the displacement in
      | x and y and the yaw angle could be
      | developed to discribe the car movement
      | in the horizontal plan
  note: in each one of these three blocks
      | only devision by mass or inertia
      | then integration is to be applied
      | as the force was derived and
      | transformed purely  to the CG
  Force_acting_on_CG_in_x : Inport
  Force_acting_on_CG_in_y : Inport  Port=2
  Moment _about _Z_axis : Inport  Port=3
  vx[m|s] : Inport  Port=4
  Beta_Slip_Angle_calculation : Subsystem
  Terminator : Terminator
  about_z_axis : Subsystem
  in_x_direction : Subsystem
  in_y_direction : Subsystem
  reset : Subsystem
  reset1 : Subsystem
  Longitudinal_velocity_Vx : Outport
  Lateral_velocity_Vy_relative_to_car : Outport  Port=2
  "yaw " : Outport  Port=3
  Displacement_y_relative_to_car : Outport  Port=4
  Displacement_x_relative_to_car : Outport  Port=5
  Beta_Slip_Angle : Outport  Port=6
  ACC_x_relative_to_car : Outport  Port=7
  ACC_Y_relative_to_car : Outport  Port=8
  Yaw_rate_of_change : Outport  Port=9
  absolute_velocity_of_car : Outport  Port=10
  wires:
  Force_acting_on_CG_in_x/1 -> in_x_direction/1(Force_acting_on_CG_in_x)
  Force_acting_on_CG_in_y/1 -> in_y_direction/1(Force_acting_on_CG_in_y)
  Moment _about _Z_axis/1 -> about_z_axis/1(Moment _about _Z_axis)
  in_x_direction/1(Longitudinal_Velocity_Vx) -> Longitudinal_velocity_Vx/1, Beta_Slip_Angle_calculation/1(Longitudinal_Velocity_Vx)
  in_x_direction/2(Displacement_x) -> Displacement_x_relative_to_car/1
  in_x_direction/3(Acceleration_Ax) -> ACC_x_relative_to_car/1
  in_y_direction/3(Acceleration_Ay) -> ACC_Y_relative_to_car/1
  in_y_direction/2(Displacement_y) -> Displacement_y_relative_to_car/1
  Beta_Slip_Angle_calculation/1(Beta_Slip_Angle) -> Beta_Slip_Angle/1
  Beta_Slip_Angle_calculation/2(absolute_velocity_of_car_with_direction) -> absolute_velocity_of_car/1
  about_z_axis/3(Yaw_angle_(rad)) -> "yaw "/1
  about_z_axis/2(Yaw_angle_Velcity) -> Yaw_rate_of_change/1
  about_z_axis/1(Yaw_Angular_ACC) -> Terminator/1
  in_y_direction/1(Lateral_Velocity_Vy) -> Lateral_velocity_Vy_relative_to_car/1, Beta_Slip_Angle_calculation/2(Longitudinal_Velocity_Vy)
  vx[m|s]/1 -> reset/1(In1), reset1/1(In1)
  reset/1(Out1) -> about_z_axis/2(reset)
  reset1/1(Out1) -> in_y_direction/2(reset)

== system PC_Simulator_Lib/Vehicle dynamics/Output_Maping ==
  Velocity_Wheels_X[m|s] : Inport
  Velocity_Wheels_Y[m|s] : Inport  Port=2
  Force_Suspention : Inport  Port=3
  Vx_COG[m|s] : Inport  Port=4
  Vy_COG[m|s] : Inport  Port=5
  ax_COG[m|s2] : Inport  Port=6
  Wheel_FL_Steering_Angle[rad] : Inport  Port=7
  Wheel_FR_Steering_Angle[rad] : Inport  Port=8
  position_CoG_Global_Vector[m] : Inport  Port=9
  Oriantation_CoG_Vector[rad] : Inport  Port=10
  Yaw_Rate[rad|s] : Inport  Port=11
  Wheel_Steering_Angle_Left[rad] : Inport  Port=12
  Wheel_Steering_Angle_Right[rad] : Inport  Port=13
  Bus Creator : BusCreator  Inputs=2
  Bus Creator2 : BusCreator  Inputs=11
  Subsystem1 : Subsystem
  Velocity_Wheels_Maping_Block : Subsystem
  Vehicle_Dynamics : Outport
  wires:
  Velocity_Wheels_Maping_Block/1(Velocity_Wheels[m|s]) -> Bus Creator2/1
  Subsystem1/1(Fz_Wheel[N]) -> Bus Creator2/2  "Fz_Wheel"
  Bus Creator/1 -> Bus Creator2/6  "Wheel_angle[rad]"
  Force_Suspention/1 -> Subsystem1/1(Force_Suspention)
  Vx_COG[m|s]/1 -> Bus Creator2/3
  Velocity_Wheels_X[m|s]/1 -> Velocity_Wheels_Maping_Block/1(Velocity_Wheels_X[m|s])
  Velocity_Wheels_Y[m|s]/1 -> Velocity_Wheels_Maping_Block/2(Velocity_Wheels_Y[m|s])
  Bus Creator2/1 -> Vehicle_Dynamics/1  "Vehicle_Dynamics"
  position_CoG_Global_Vector[m]/1 -> Bus Creator2/7
  Oriantation_CoG_Vector[rad]/1 -> Bus Creator2/8
  Wheel_FL_Steering_Angle[rad]/1 -> Bus Creator/1
  Wheel_FR_Steering_Angle[rad]/1 -> Bus Creator/2
  ax_COG[m|s2]/1 -> Bus Creator2/5  "ax_COG[m|s2]"
  Vy_COG[m|s]/1 -> Bus Creator2/4  "Vy_COG[m|s]"
  Yaw_Rate[rad|s]/1 -> Bus Creator2/9  "Yaw_Rate[rad|s]"
  Wheel_Steering_Angle_Left[rad]/1 -> Bus Creator2/10  "Wheel_Steering_Angle_Left[rad]"
  Wheel_Steering_Angle_Right[rad]/1 -> Bus Creator2/11  "Wheel_Steering_Angle_Right[rad]"

== system PC_Simulator_Lib/Vehicle dynamics/Vertical_Dyn. ==
  Vertical_Force_CG : Inport
  Moment_X-axis_CG : Inport  Port=2
  Moment_Y-axis_CG : Inport  Port=3
  Mass*gravity_in_Z : Inport  Port=4
  Z0 : Inport  Port=5
  Invers_Trangnometric_conv : Subsystem
  Mass_Distribution : Subsystem
  Trangnometric_conv : Subsystem
  Vertical_movement : Subsystem
  suspention_System : Subsystem
  Vertical_Displacement_Z_CG : Outport
  Vertical_Displacement_Z_vehicle_corners(4) : Outport  Port=2
  pitch : Outport  Port=3
  Roll : Outport  Port=4
  Force_Suspention(4) : Outport  Port=5
  Length_Suspention(4) : Outport  Port=6
  Z1(4) : Outport  Port=7
  Vertical_Velocity_Z_CG[m|s] : Outport  Port=8
  wires:
  Invers_Trangnometric_conv/3(Pitch_actual) -> pitch/1
  Vertical_Force_CG/1 -> Vertical_movement/1(Vertical_Force_CG)
  Moment_Y-axis_CG/1 -> Vertical_movement/2(Moment_Y-axis_CG)
  Moment_X-axis_CG/1 -> Vertical_movement/3(Moment_X-axis_CG)
  Vertical_movement/1(Vertical_Displacement_Z_CG) -> Trangnometric_conv/1(Vertical_Displacement_Z_CG)
  Vertical_movement/2(Pitch) -> Trangnometric_conv/2(Pitch)
  Vertical_movement/3(Roll) -> Trangnometric_conv/3(Roll)
  suspention_System/1(Force_Suspention(4)) -> Force_Suspention(4)/1
  suspention_System/2(Hight_Suspention(4)) -> Length_Suspention(4)/1
  Mass_Distribution/1(Forces_Z_Mass) -> suspention_System/3(intial_force_from_mass_Wheels(4))
  Z0/1 -> suspention_System/2(Vertical_Displacement_Z0(4))
  suspention_System/3(Z1(4)) -> Z1(4)/1
  suspention_System/4(Vertical_Displacement_Z_vehicle_corners_actual(4)) -> Invers_Trangnometric_conv/1(Vertical_Displacement_Z_vehicle_corners_actual(4)), Vertical_Displacement_Z_vehicle_corners(4)/1
  Invers_Trangnometric_conv/1(Vertical_Displacement_Z_CG_actual) -> Vertical_Displacement_Z_CG/1
  Invers_Trangnometric_conv/2(Roll_actual) -> Roll/1
  Mass*gravity_in_Z/1 -> Mass_Distribution/1(Mass*gravity_in_Z)
  Trangnometric_conv/1(Vertical_Displacement_Z_vehicle_corners(4)) -> suspention_System/1(Vertical_Displacement_Z2_vehicle_corners(4))
  Vertical_movement/4(Vertical_Velocity_Z_CG[m|s]) -> Vertical_Velocity_Z_CG[m|s]/1

== system PC_Simulator_Lib/Vehicle dynamics/force_from_wheel_cordination_transformation ==
  note: this block is to analyze the
      | forces acting on the wheels
      |  coordination to find thier
      | components on the car coordination
      | -with respect to CAR XY-
      | and provides the angle of rotation
      | of each wheel due to ackermann
  steering_Angle_HMI_in_range[-1 1] : Inport
  force_from_wheel_fornt_left_in_x_relative_to_tire : Inport  Port=2
  force_from_wheel_fornt_right_in_x_relative_to_tire : Inport  Port=3
  force_from_wheel_rear_left_in_x_relative_to_tire : Inport  Port=4
  force_from_wheel_rear_right_in_x_relative_to_tire : Inport  Port=5
  force_from_wheel_fornt_left_in_y_relative_to_tire : Inport  Port=6
  force_from_wheel_fornt_right_in_y_relative_to_tire : Inport  Port=7
  force_from_wheel_rear_left_in_y_relative_to_tire : Inport  Port=8
  force_from_wheel_rear_right_in_y_relative_to_tire : Inport  Port=9
  Mux : Mux
  Mux1 : Mux
  Steer_model : Subsystem
  Forces_on_x_from_wheel_mux(4) : Outport
  Forces_on_y_from_wheel_mux(4) : Outport  Port=2
  angle_of_rotation_of_front_left_wheel : Outport  Port=3
  angle_of_rotation_of_front_right_wheel : Outport  Port=4
  wires:
  force_from_wheel_fornt_left_in_x_relative_to_tire/1 -> Steer_model/2(FLx_T)
  force_from_wheel_fornt_right_in_x_relative_to_tire/1 -> Steer_model/3(FRx_T)
  force_from_wheel_fornt_left_in_y_relative_to_tire/1 -> Steer_model/4(FLy_T)
  force_from_wheel_fornt_right_in_y_relative_to_tire/1 -> Steer_model/5(FRy_T)
  Steer_model/1(FLx) -> Mux/1
  Steer_model/2(FRx) -> Mux/2
  force_from_wheel_rear_left_in_x_relative_to_tire/1 -> Mux/3
  force_from_wheel_rear_right_in_x_relative_to_tire/1 -> Mux/4
  Steer_model/4(FRy) -> Mux1/2
  Steer_model/3(FLy) -> Mux1/1
  force_from_wheel_rear_left_in_y_relative_to_tire/1 -> Mux1/3
  force_from_wheel_rear_right_in_y_relative_to_tire/1 -> Mux1/4
  Mux/1 -> Forces_on_x_from_wheel_mux(4)/1
  Mux1/1 -> Forces_on_y_from_wheel_mux(4)/1
  Steer_model/5(FL_Angle) -> angle_of_rotation_of_front_left_wheel/1
  Steer_model/6(FR_Angle) -> angle_of_rotation_of_front_right_wheel/1
  steering_Angle_HMI_in_range[-1 1]/1 -> Steer_model/1(Steering_Angle_HMI_[-1 1])

== system PC_Simulator_Lib/Vehicle dynamics/velocity ==
  longitudenal_velocity_Vx : Inport
  Lateral_velocity_Vy : Inport  Port=2
  rate_of_change_Yaw_Angle : Inport  Port=3
  angel_of_rotation_of_front_left_wheel : Inport  Port=4
  angel_of_rotation_of_front_Right_wheel : Inport  Port=5
  Mux2 : Mux
  Mux3 : Mux
  R : Subsystem
  to_tire : Subsystem
  velocity_at_Front_Left : Subsystem
  velocity_at_Front_Right : Subsystem
  velocity_at_Rear_Left : Subsystem
  velocity_at_Rear_Right : Subsystem
  velocity_conditioning : Subsystem
  velocity_at_wheels_in_X_mux(4) : Outport
  velocity_at_wheels_in_Y_mux(4) : Outport  Port=2
  R_CG : Outport  Port=3
  wires:
  rate_of_change_Yaw_Angle/1 -> velocity_at_Front_Left/1(rate_of_change_Yaw_Angle), velocity_at_Rear_Left/1(rate_of_change_Yaw_Angle), velocity_at_Rear_Right/1(rate_of_change_Yaw_Angle), velocity_at_Front_Right/1(rate_of_change_Yaw_Angle)
  longitudenal_velocity_Vx/1 -> velocity_at_Front_Left/2(longitudenal_velocity_Vx), velocity_at_Rear_Left/2(longitudenal_velocity_Vx), velocity_at_Rear_Right/2(longitudenal_velocity_Vx), R/2(longitudenal_velocity_Vx), velocity_at_Front_Right/2(longitudenal_velocity_Vx), velocity_conditioning/4(VxCG)
  velocity_at_Front_Left/1(velocity_at_Front_left_in_X) -> Mux2/1
  velocity_at_Front_Right/1(velocity_at_Front_Right_in_X) -> Mux2/2
  velocity_at_Rear_Left/1(velocity_at_Rear_left_in_X) -> Mux2/3
  velocity_at_Rear_Right/1(velocity_at_Rear_Right_in_X) -> Mux2/4
  velocity_at_Front_Right/2(velocity_at_Front_Right_in_Y) -> Mux3/2
  velocity_at_Front_Left/2(velocity_at_Front_left_in_Y) -> Mux3/1
  velocity_at_Rear_Left/2(velocity_at_Rear_left_in_Y) -> Mux3/3
  velocity_at_Rear_Right/2(velocity_at_Rear_Right_in_Y) -> Mux3/4
  velocity_at_Rear_Left/3(slip_angel_at_Rear_left) -> R/1(slip_angel_at_Rear_left)
  Lateral_velocity_Vy/1 -> velocity_at_Front_Left/3(Lateral_velocity_Vy), velocity_at_Rear_Left/3(Lateral_velocity_Vy), velocity_at_Rear_Right/3(Lateral_velocity_Vy), R/3(Lateral_velocity_Vy), velocity_at_Front_Right/3(Lateral_velocity_Vy), velocity_conditioning/5(VyCG)
  R/1(R_CG) -> velocity_conditioning/3(R_CGin)
  Mux3/1 -> velocity_conditioning/2(velocity_at_wheels_in_Y_mux(4)in)
  Mux2/1 -> velocity_conditioning/1(velocity_at_wheels_in_X_mux(4)in)
  velocity_conditioning/2(velocity_at_wheels_in_Y_mux(4)out) -> to_tire/4(velocity_at_wheels_in_Y_mux(4))
  velocity_conditioning/1(velocity_at_wheels_in_X_mux(4)out) -> to_tire/3(velocity_at_wheels_in_X_mux(4))
  angel_of_rotation_of_front_left_wheel/1 -> to_tire/1(angel_of_rotation_of_front_left_wheel)
  angel_of_rotation_of_front_Right_wheel/1 -> to_tire/2(angel_of_rotation_of_front_Right_wheel)
  to_tire/1(velocity_at_wheels_in_X_mux(4)final) -> velocity_at_wheels_in_X_mux(4)/1
  to_tire/2(velocity_at_wheels_in_Y_mux(4)final) -> velocity_at_wheels_in_Y_mux(4)/1
  velocity_conditioning/3(R_CGout) -> R_CG/1

== system PC_Simulator_Lib/Vehicle dynamics/xy_Global ==
  note: yaw_vehicle
  Vx_CG : Inport
  Vy_CG : Inport  Port=2
  rate_of_change_Yaw_Angle : Inport  Port=3
  Add8 : Sum  Inputs=+-
  Add9 : Sum
  Integrator1 : Integrator  InitialCondition=Heading_init
  Integrator8 : Integrator  InitialCondition=X_init
  Integrator9 : Integrator  InitialCondition=Y_init
  Product{16..19} (4 alike) : Product  RndMeth=Zero
  Trigonometric Function : Trigonometry  Operator=cos
  Trigonometric Function1 : Trigonometry
  Vx_global : Outport
  Vy_global : Outport  Port=2
  x_CG : Outport  Port=3
  y_CG : Outport  Port=4
  Actual_YAW : Outport  Port=5
  wires:
  Trigonometric Function1/1 -> Product18/2, Product17/2
  Trigonometric Function/1 -> Product16/2, Product19/1
  Integrator9/1 -> y_CG/1
  Product18/1 -> Add9/1
  Product19/1 -> Add9/2
  Product17/1 -> Add8/2
  Product16/1 -> Add8/1
  Add8/1 -> Integrator8/1, Vx_global/1
  Vy_CG/1 -> Product19/2, Product17/1
  Vx_CG/1 -> Product18/1, Product16/1
  Integrator1/1 -> Actual_YAW/1, Trigonometric Function/1, Trigonometric Function1/1
  rate_of_change_Yaw_Angle/1 -> Integrator1/1
  Integrator8/1 -> x_CG/1
  Add9/1 -> Integrator9/1, Vy_global/1

== system PC_Simulator_Lib/ADAS/Decision_Making_ADAS/Decision_Unit ==
  Active_System : Inport
  Set_Speed_User[m|s] : Inport  Port=2
  Time_Gap_User[s] : Inport  Port=3
  Object_Inlane[bool] : Inport  Port=4
  Distance_2_Object_Sensor[m] : Inport  Port=5
  v_relative_Sensor[m|s] : Inport  Port=6
  T_current[m] : Inport  Port=7
  Direction_delta_T_Available : Inport  Port=8
  Lateral_Distance_Available[m] : Inport  Port=9
  Heading_Angle_Difference_absolute[deg] : Inport  Port=10
  velocity_VUT[m|s] : Inport  Port=11
  Clock : Clock
  Compare To Constant : simulink/Logic and Bit Operations/Compare To Constant  relop===  const=3.0  OutDataTypeStr=boolean
  Compare To Constant1 : simulink/Logic and Bit Operations/Compare To Constant  relop===  const=4  OutDataTypeStr=boolean
  Data Type Conversion : DataTypeConversion
  Logical Operator : Logic  Operator=OR  AllPortsSameDT=off  OutDataTypeStr=boolean
  Memory : Memory
  Product : Product
  S-Function : S-Function  FunctionName=DecisionUnit  EnableBusSupport=off
  Saturation : Saturate  UpperLimit=inf  LowerLimit=0
  critical_Braking_distance_determination : Subsystem
  Enable_Longitudinal_Controller[bool] : Outport
  Enable_Lateral_Controller[bool] : Outport  Port=2
  Velocity_desired_Free_Driving[m|s] : Outport  Port=3
  Object_in_Lane[bool] : Outport  Port=4
  Distance_2_Object[m] : Outport  Port=5
  v_relative[m|s] : Outport  Port=6
  Time_Gap[s] : Outport  Port=7
  T_desird[m] : Outport  Port=8
  Lateral_Velocity_Max[m|s] : Outport  Port=9
  Acceleration_Velocity_Control_Switching[0 1] : Outport  Port=10
  a_x_desiredm|s2] : Outport  Port=11
  level_of_danger_front[0-3] : Outport  Port=12
  Brake_distance[m] : Outport  Port=13
  wires:
  Memory/1 -> v_relative[m|s]/1
  Saturation/1 -> Brake_distance[m]/1
  Data Type Conversion/1 -> Product/2
  Logical Operator/1 -> Data Type Conversion/1
  Compare To Constant1/1 -> Logical Operator/2
  Compare To Constant/1 -> Logical Operator/1
  Product/1 -> Saturation/1
  S-Function/12 -> level_of_danger_front[0-3]/1
  velocity_VUT[m|s]/1 -> S-Function/13
  S-Function/4 -> Object_in_Lane[bool]/1
  Time_Gap_User[s]/1 -> S-Function/3
  Object_Inlane[bool]/1 -> S-Function/4
  S-Function/6 -> Memory/1
  v_relative_Sensor[m|s]/1 -> S-Function/6, critical_Braking_distance_determination/1(v_relative_Sensor[m|s])
  S-Function/7 -> Time_Gap[s]/1
  Distance_2_Object_Sensor[m]/1 -> S-Function/5
  S-Function/1 -> Enable_Longitudinal_Controller[bool]/1
  S-Function/2 -> Enable_Lateral_Controller[bool]/1
  S-Function/5 -> Distance_2_Object[m]/1
  S-Function/3 -> Velocity_desired_Free_Driving[m|s]/1
  S-Function/8 -> T_desird[m]/1
  S-Function/9 -> Lateral_Velocity_Max[m|s]/1
  Active_System/1 -> S-Function/1, Compare To Constant/1, Compare To Constant1/1
  Set_Speed_User[m|s]/1 -> S-Function/2
  T_current[m]/1 -> S-Function/7
  S-Function/11 -> a_x_desiredm|s2]/1
  S-Function/10 -> Acceleration_Velocity_Control_Switching[0 1]/1
  critical_Braking_distance_determination/1(Braking_Distance[m]) -> S-Function/8, Product/1
  Direction_delta_T_Available/1 -> S-Function/9
  Lateral_Distance_Available[m]/1 -> S-Function/10
  Heading_Angle_Difference_absolute[deg]/1 -> S-Function/11
  Clock/1 -> S-Function/12
